simulink model "FIR_FILTER_CASCADEFORM_7"  (R2020b)
settings: Solver=VariableStepAuto  StartTime=0.0  StopTime=10.0  RelTol=1e-3
settings Model: Creator=intel  LastModifiedBy=intel

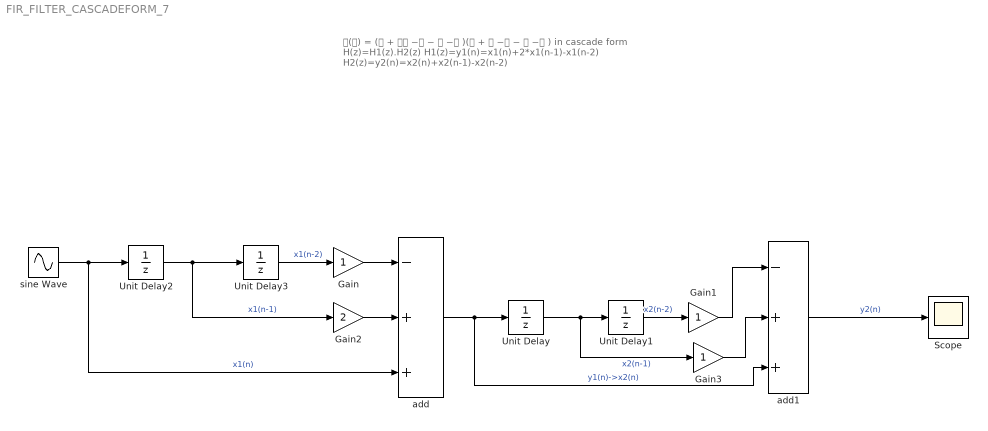
== system FIR_FILTER_CASCADEFORM_7 ==
  note: 𝐇(𝐳) = (𝟏 + 𝟐𝐳 −𝟏 − 𝐳 −𝟐 )(𝟏 + 𝐳 −𝟏 − 𝐳 −𝟐 )
      | in cascade form H(z)=H1(z).H2(z)
      | H1(z)=y1(n)=x1(n)+2*x1(n-1)-x1(n-2)
      | H2(z)=y2(n)=x2(n)+x2(n-1)-x2(n-2)
  Gain : Gain
  Gain1 : Gain
  Gain2 : Gain  Gain=2
  Gain3 : Gain
  Scope : Scope
  Unit Delay{,1..3} (4 alike) : UnitDelay  SampleTime=-1  HasFrameUpgradeWarning=on
  add : Sum  Inputs=-++
  add1 : Sum  Inputs=-++
  sine Wave : Sin  SampleTime=0
  wires:
  sine Wave/1 -> Unit Delay2/1, add/3  "x1(n)"
  Gain2/1 -> add/2
  Gain/1 -> add/1
  Unit Delay2/1 -> Unit Delay3/1, Gain2/1  "x1(n-1)"
  Unit Delay3/1 -> Gain/1  "x1(n-2)"
  Unit Delay/1 -> Gain3/1, Unit Delay1/1  "x2(n-1)"
  add/1 -> Unit Delay/1, add1/3  "y1(n)->x2(n)"
  Unit Delay1/1 -> Gain1/1  "x2(n-2)"
  Gain1/1 -> add1/1
  add1/1 -> Scope/1  "y2(n)"
  Gain3/1 -> add1/2
